simulink model "gm_lab2_first_part"  (R2022a)
settings: Solver=VariableStepAuto  StartTime=0.0  StopTime=10.0  RelTol=1e-3
settings Model: Creator=Даниил  LastModifiedBy=Даниил
settings OptimizationCC: BlockReduction=off  ConditionallyExecuteInputs=off
settings DebuggingCC: InheritedTsInSrcMsg=none

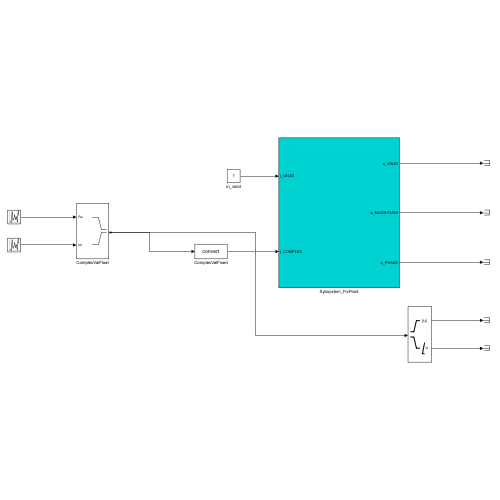
[thumbnail: Simulink's stored preview of the top-level diagram]
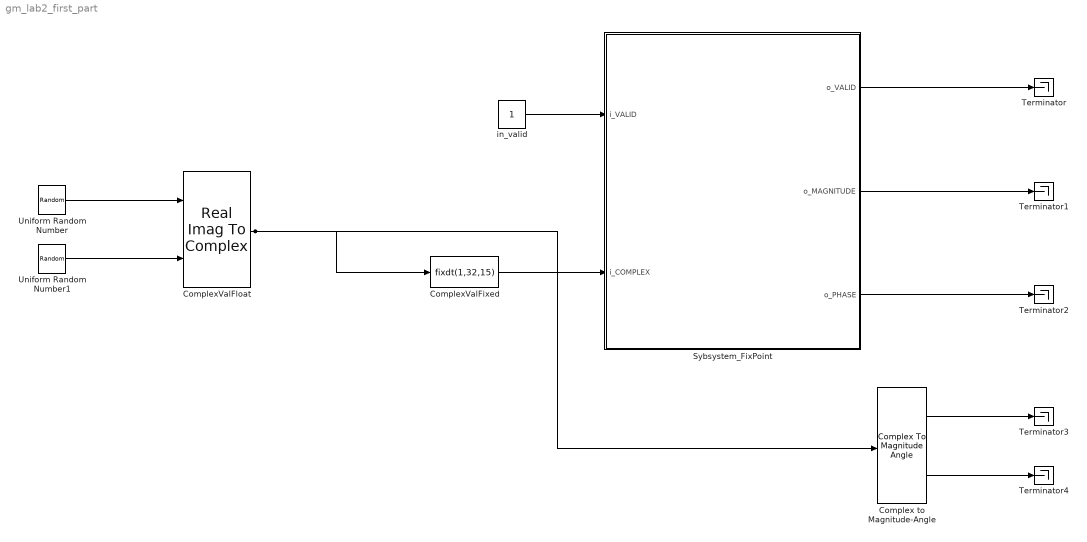
== system gm_lab2_first_part ==
  Complex to Magnitude-Angle : ComplexToMagnitudeAngle
  ComplexValFixed : DataTypeConversion  OutDataTypeStr=fixdt(1,32,15)  RndMeth=Round  SaturateOnIntegerOverflow=off
  ComplexValFloat : RealImagToComplex
  Sybsystem_FixPoint : Subsystem
  Terminator{,1..4} (5 alike) : Terminator
  Uniform Random Number : UniformRandomNumber  Minimum=-2 ^(17 - 1)  Maximum=2 ^(17-1) - 1  Seed=17  SampleTime=1
  Uniform Random Number1 : UniformRandomNumber  Minimum=-2 ^(17 - 1)  Maximum=2 ^(17-1) - 1  Seed=18  SampleTime=1
  in_valid : Constant  OutDataTypeStr=boolean  SampleTime=1
  wires:
  Sybsystem_FixPoint/1(o_VALID) -> Terminator/1
  Uniform Random Number/1 -> ComplexValFloat/1
  Uniform Random Number1/1 -> ComplexValFloat/2
  Sybsystem_FixPoint/2(o_MAGNITUDE) -> Terminator1/1
  Sybsystem_FixPoint/3(o_PHASE) -> Terminator2/1
  Complex to Magnitude-Angle/2 -> Terminator4/1
  Complex to Magnitude-Angle/1 -> Terminator3/1
  ComplexValFloat/1 -> ComplexValFixed/1, Complex to Magnitude-Angle/1
  in_valid/1 -> Sybsystem_FixPoint/1(i_VALID)
  ComplexValFixed/1 -> Sybsystem_FixPoint/2(i_COMPLEX)

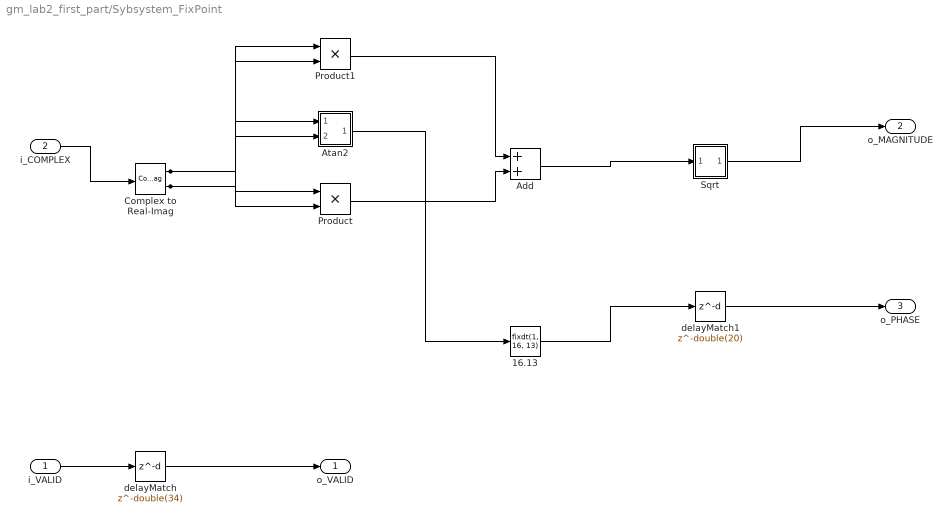
== system gm_lab2_first_part/Sybsystem_FixPoint ==
  i_VALID : Inport  OutDataTypeStr=boolean  PortDimensions=1  SampleTime=1
  i_COMPLEX : Inport  Port=2  OutDataTypeStr=fixdt(1, 32, 15)  PortDimensions=1  SampleTime=1
      settings: SignalType=complex
  16.13 : DataTypeConversion  OutDataTypeStr=fixdt(1, 16, 13)  RndMeth=Round  SampleTime=1  SaturateOnIntegerOverflow=off
  Add : Sum  AccumDataTypeStr=fixdt(1, 64, 30)  OutDataTypeStr=fixdt(1, 64, 30)  SampleTime=1
  Atan2 : Subsystem
  Complex to Real-Imag : ComplexToRealImag  SampleTime=1
  Product : Product  Inputs=**  OutDataTypeStr=fixdt(1, 64, 30)  SampleTime=1
  Product1 : Product  Inputs=**  OutDataTypeStr=fixdt(1, 64, 30)  SampleTime=1
  Sqrt : Subsystem
  delayMatch : Delay  DelayLength=double(34)  InitialCondition=0  SampleTime=1
  delayMatch1 : Delay  DelayLength=double(20)  InitialCondition=0  SampleTime=1
  o_VALID : Outport  SampleTime=1
  o_MAGNITUDE : Outport  Port=2  SampleTime=1
  o_PHASE : Outport  Port=3  SampleTime=1
  wires:
  delayMatch/1 -> o_VALID/1
  i_COMPLEX/1 -> Complex to Real-Imag/1
  delayMatch1/1 -> o_PHASE/1
  Add/1 -> Sqrt/1(In1)
  Atan2/1(Out1) -> 16.13/1
  Complex to Real-Imag/1 -> Product1/2, Product1/1, Atan2/2(In2)
  Complex to Real-Imag/2 -> Product/2, Product/1, Atan2/1(In1)
  Product/1 -> Add/2
  Product1/1 -> Add/1
  Sqrt/1(Out1) -> o_MAGNITUDE/1
  i_VALID/1 -> delayMatch/1
  16.13/1 -> delayMatch1/1

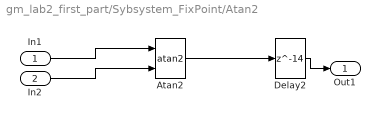
== system gm_lab2_first_part/Sybsystem_FixPoint/Atan2 ==
  In1 : Inport
  In2 : Inport  Port=2
  Atan2 : Trigonometry  Operator=atan2  ApproximationMethod=CORDIC
  Delay2 : Delay  DelayLength=14
  Out1 : Outport
  wires:
  In1/1 -> Atan2/1
  In2/1 -> Atan2/2
  Atan2/1 -> Delay2/1
  Delay2/1 -> Out1/1

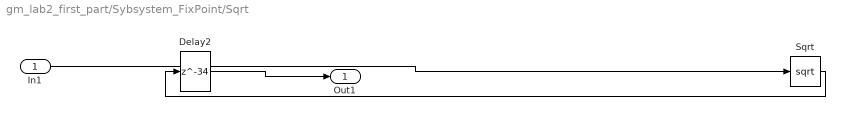
== system gm_lab2_first_part/Sybsystem_FixPoint/Sqrt ==
  In1 : Inport
  Delay2 : Delay  DelayLength=34
  Sqrt : Sqrt  OutDataTypeStr=fixdt(1,33,15)
  Out1 : Outport
  wires:
  In1/1 -> Sqrt/1
  Sqrt/1 -> Delay2/1
  Delay2/1 -> Out1/1
